simulink model "Project_VirtualWall_V7"  (R2014a)
settings: Solver=FixedStepDiscrete  StartTime=0.0  StopTime=inf  FixedStep=0.0002  RelTol=1e-3
PreLoadFcn:
  | SampleTime = 0.0002;
  | 
  | omega_set = Simulink.Signal;
  | omega_set.Description = ' Omega control set parameter (for read)';
  | omega_set.DataType = 'double';
  | omega_set.Complexity = 'real';
  | omega_set.Dimensions = 9;
  | omega_set.SamplingMode = 'Sample based';
  | omega_set.SampleTime = SampleTime;
  | omega_set.InitialValue = '[0 0 0 0 0 0 0 0 0] ';
undefined symbols (not defined in the file or in its folder): mdionipcie
libraries: slrtlib x16, simulink x9, dsparch4 x6, simulink_extras x3, phantom_kinematics_lib x2, dspmtrx3 x2, dspswit3 x1
settings Model: SimulationMode=external  BufferReuse=off  Creator=janezp  LastModifiedBy=student
settings SolverCC: EnableConcurrentExecution=on
settings DataIOCC: LimitDataPoints=off  MaxDataPoints=5000000  SaveFormat=Structure  SignalLogging=off  SaveTime=off
settings OptimizationCC: BlockReduction=off  OptimizeBlockIOStorage=off  BufferReuse=off  GlobalBufferReuse=off  ExpressionFolding=off  ExpressionDepthLimit=2147483647  LocalBlockOutputs=off  InitFltsAndDblsToZero=on
settings DebuggingCC: SaveWithParameterizedLinksMsg=none  MergeDetectMultiDrivingBlocksExec=error  SignalResolutionControl=TryResolveAllWithWarning  InheritedTsInSrcMsg=none  MultiTaskDSMMsg=warning  MultiTaskCondExecSysMsg=none  UnconnectedInputMsg=none  UnconnectedOutputMsg=none  UnconnectedLineMsg=none  StateNameClashWarn=warning
settings HardwareCC: ProdIntDivRoundTo=Zero  ProdEndianess=LittleEndian  ProdHWDeviceType=Generic->32-bit x86 compatible
settings SFSimCC: SimParseCustomCode=off
settings RTWCC: SystemTargetFile=slrt.tlc  TemplateMakefile=slrt_default_tmf  Description=Simulink Real-Time  ProcessScript=slrt_make_rtw_hook  CustomInclude="\"C:\\Program Files (x86)\\MATLAB\\R2014a\\toolbox\\robotica\\haptics\\collisiondetection\\\""  IncludeERTFirstTime=on  RTWCompilerOptimization=On
settings RTWCC: CustomLibrary=|
  | \..\..\math\mathlib.lib
  | deBug.obj
settings SimulinkRealTimeCC: GeneratePreprocessorConditionals=Disable all  EnableShiftOperators=on  RL32LogBufSizeModifier=5000000

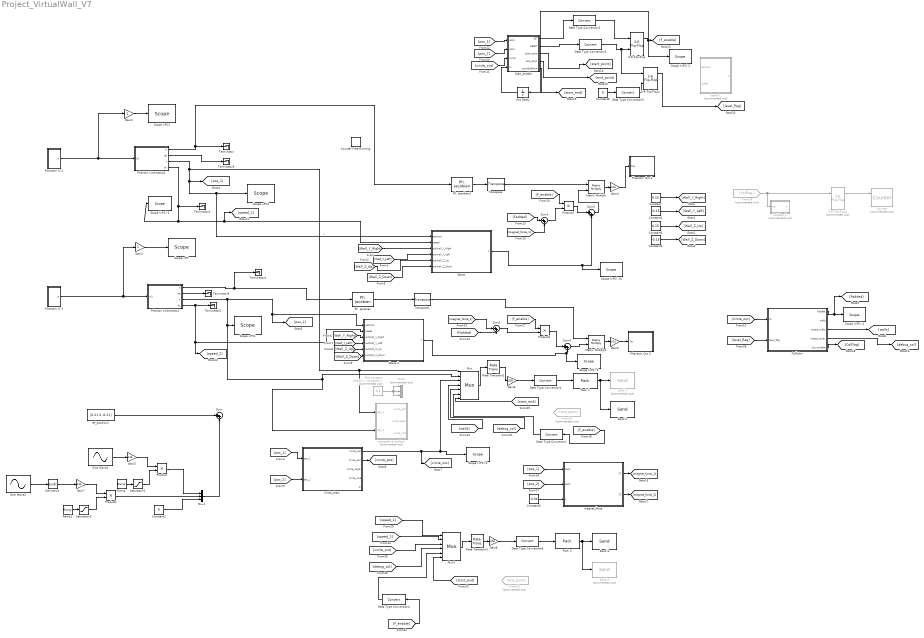
== system Project_VirtualWall_V7 ==
  "Circle_draw " : MATLAB Function  TreatAsAtomicUnit=on
  "Collision " : MATLAB Function  TreatAsAtomicUnit=on
  Collision 1 : MATLAB Function  Commented=on  TreatAsAtomicUnit=on
  Constant : Constant  Value=0.15
  Constant1 : Constant  Value=-0.15
  Constant2 : Constant  Value=0  OutDataTypeStr=double  SampleTime=-1
  Constant3 : Constant  Value=0.15
  Constant4 : Constant  Value=-0.15
  Constant5 : Constant  Value=0.04
  Constant6 : Constant  Value=0
  Counter : dspswit3/Counter  Commented=on  Direction=Up  CountEvent=Rising edge  CounterSize=User defined  MaxCount=255  InitialCount=0  Output=Count and Hit  HitValue=32  ResetInput=on  SamplesPerFrame=1  Ts=1  CntDtype=double  HitDtype=Logical
  Counter Free-Running : simulink/Sources/Counter Free-Running  NumBits=16  tsamp=-1
  Data Type Conversion{,1..6} (7 alike) : DataTypeConversion
  Derivative : Derivative
  From24 : From  Commented=on  GotoTag=ColFlag
  From26 : From  Commented=on  GotoTag=end_point
  From33 : From  Commented=on  GotoTag=end_point
  Gain1 : Gain
  Gain2 : Gain
  Gain3 : Gain  Gain=0.05
  Gain4 : Gain  Gain=0.15
  Gain5 : Gain  Gain=0.15
  Gain6 : Gain  Gain=100
  Gain7 : Gain  Gain=0.05
  Gain8 : Gain  Gain=100
  Matrix Multiply : Product  Multiplication=Matrix(*)
  Matrix Multiply1 : Product  Multiplication=Matrix(*)
  Mux : Mux  Inputs=7
  Mux1 : Mux  Inputs=3
  Mux2 : Mux  Commented=on  Inputs=3
  Mux3 : Mux  Inputs=6
  Pack 1 : slrtlib/UDP/Pack   datatypes={'single'}  byteAlign=1
  Pack 2 : slrtlib/UDP/Pack   datatypes={'single'}  byteAlign=1
  Ph. Jacobian : phantom_kinematics_lib/Ph. Jacobian
  Ph. Jacobian1 : phantom_kinematics_lib/Ph. Jacobian
      link override phantomJacobian: FunctionName=phantomJacobian  SFunctionModules=phantomJacobian_wrapper
  Phantom In 2 : Subsystem  mask(Phantom Input){channel=3, sampletime=0.0002, slot=[2,3], phantomid=Phantom ONE}
      mask prompts: channel "Number of joints:"; sampletime "Sample time:"; slot "PCI slot (-1: autosearch):"; phantomid "Phantom ID:"
      mask help: Block output is a vector of Phantom joint angles.
      mask init:
      | set_param(gcb', 'LinkStatus', 'none')
      | current_block = gcb;
      | 
      | line = find_system(current_block, 'LookUnderMasks', 'on', 'FindAll', 'on', 'type', 'line');
      | for ii=1:length(line)
      |     delete_line(line(ii));
      | end
      | 
      | set_param([current_block,'/Phantom Input'], 'channel', num2str(channel));
      | set_param([current_block,'/Phantom Input'], 'sampletime', sampletime);
      | set_param([current_block,'/Phantom Input'], 'slot', slot);
      | set_param([current_block,'/Phantom Input'], 'phantomid', num2str(phantomid-1));
      | 
      | set_param([current_block,'/Mux'], 'Inputs', int2str(channel)); 
      | 
      | add_line(current_block, 'Mux/1', 'q/1'); 
      | 
      | for i=1:channel,
      |     add_line(current_block, ['Phantom Input/', int2str(i)], ['Mux/', int2str(i)]); 
      | end
      mask TypeOptions phantomid: Phantom ONE | Phantom TWO | Phantom THREE
  Phantom In 3 : Subsystem  mask(Phantom Input){channel=3, sampletime=0.0002, slot=[4,0], phantomid=Phantom TWO}
      mask prompts: channel "Number of joints:"; sampletime "Sample time:"; slot "PCI slot (-1: autosearch):"; phantomid "Phantom ID:"
      mask help: Block output is a vector of Phantom joint angles.
      mask init: same as Project_VirtualWall_V7/Phantom In 2
      mask TypeOptions phantomid: Phantom ONE | Phantom TWO | Phantom THREE
  Phantom Out 2 : Subsystem  mask(Phantom Output){sampletime=0.0002, slot=[2,3]}
      mask prompts: sampletime "Sample time:"; slot "PCI slot (-1: autosearch):"
      mask help: Input is torque vector for Phantom motors.
      mask init:
      | set_param(gcb', 'LinkStatus', 'none')
      | current_block = gcb;
      | 
      | set_param([current_block,'/Phantom Output'], 'sampletime', sampletime);
      | set_param([current_block,'/Phantom Output'], 'slot', slot);
  Phantom Out 3 : Subsystem  mask(Phantom Output){sampletime=0.0002, slot=[4,0]}
      mask prompts: sampletime "Sample time:"; slot "PCI slot (-1: autosearch):"
      mask help: Input is torque vector for Phantom motors.
      mask init:
      | set_param(gcb', 'LinkStatus', 'none')
      | current_block = gcb;
      | 
      | set_param([current_block,'/Phantom Output'], 'sampletime', sampletime);
      | set_param([current_block,'/Phantom Output'], 'slot', slot);
  Phanton kinematics1 : Subsystem
  Phanton kinematics2 : Subsystem
  Product{,1..3} (4 alike) : Product
  Ramp : simulink/Sources/Ramp  slope=0.25  start=1  X0=0
  Ramp1 : simulink/Sources/Ramp  slope=0.25  start=1  X0=0
  Rate Transition1 : RateTransition  OutPortSampleTime=0.01
  Rate Transition2 : RateTransition  OutPortSampleTime=0.01
  S-R Flip-Flop : simulink_extras/Flip Flops/S-R Flip-Flop  initial_condition=0
  S-R Flip-Flop1 : simulink_extras/Flip Flops/S-R Flip-Flop  Commented=on  initial_condition=0
  S-R Flip-Flop2 : simulink_extras/Flip Flops/S-R Flip-Flop  initial_condition=0
  Saturation1 : Saturate  UpperLimit=1  LowerLimit=0
  Saturation2 : Saturate  UpperLimit=1  LowerLimit=0
  Scope (xPC) 1 : slrtlib/Displays and Logging/Scope   scopeno=6  scopetype=Target  autostart=on  viewmode=Numerical  formatstr='Tx: %15.6f, Ty: %15.6f, Tz: %15.6f'  grid=on  ylimits=[0,0]  nosamples=50  noprepostsamples=0  interleave=1  triggermode=FreeRun  triggersignal=1  trigsignalfromport=off  triggerlevel=0.0  triggerslope=Either  triggerscope=1  triggersample=0  filename=data.dat  mode=Lazy  writesize=512  autorestart=off  dynamicfilemode=off  maxwritefilesize=512*1024^2
  Scope (xPC) 10 : slrtlib/Displays and Logging/Scope   scopeno=10  scopetype=Target  autostart=on  viewmode=Numerical  formatstr='Fx1: %15.6f,Fy: %15.6f,Fz: %15.6f'  grid=on  ylimits=[0,0]  nosamples=50  noprepostsamples=0  interleave=1  triggermode=FreeRun  triggersignal=1  trigsignalfromport=off  triggerlevel=0.0  triggerslope=Either  triggerscope=1  triggersample=0  filename=data.dat  mode=Lazy  writesize=512  autorestart=off  dynamicfilemode=off  maxwritefilesize=512*1024^2
  Scope (xPC) 2 : slrtlib/Displays and Logging/Scope   scopeno=5  scopetype=Target  autostart=on  viewmode=Numerical  formatstr='Fx1: %15.6f,Fy: %15.6f,Fz: %15.6f'  grid=on  ylimits=[0,0]  nosamples=50  noprepostsamples=0  interleave=1  triggermode=FreeRun  triggersignal=1  trigsignalfromport=off  triggerlevel=0.0  triggerslope=Either  triggerscope=1  triggersample=0  filename=data.dat  mode=Lazy  writesize=512  autorestart=off  dynamicfilemode=off  maxwritefilesize=512*1024^2
  Scope (xPC) 3 : slrtlib/Displays and Logging/Scope   scopeno=7  scopetype=Target  autostart=on  viewmode=Numerical  formatstr='Fx1: %15.6f,Fy: %15.6f,Fz: %15.6f'  grid=on  ylimits=[0,0]  nosamples=50  noprepostsamples=0  interleave=1  triggermode=FreeRun  triggersignal=1  trigsignalfromport=off  triggerlevel=0.0  triggerslope=Either  triggerscope=1  triggersample=0  filename=data.dat  mode=Lazy  writesize=512  autorestart=off  dynamicfilemode=off  maxwritefilesize=512*1024^2
  Scope (xPC) 4 : slrtlib/Displays and Logging/Scope   scopeno=8  scopetype=Target  autostart=on  viewmode=Numerical  formatstr='Fx1: %15.6f,Fy: %15.6f,Fz: %15.6f'  grid=on  ylimits=[0,0]  nosamples=50  noprepostsamples=0  interleave=1  triggermode=FreeRun  triggersignal=1  trigsignalfromport=off  triggerlevel=0.0  triggerslope=Either  triggerscope=1  triggersample=0  filename=data.dat  mode=Lazy  writesize=512  autorestart=off  dynamicfilemode=off  maxwritefilesize=512*1024^2
  Scope (xPC) 5 : slrtlib/Displays and Logging/Scope   scopeno=9  scopetype=Target  autostart=on  viewmode=Numerical  formatstr='Fx1: %15.6f,Fy: %15.6f,Fz: %15.6f'  grid=on  ylimits=[0,0]  nosamples=50  noprepostsamples=0  interleave=1  triggermode=FreeRun  triggersignal=1  trigsignalfromport=off  triggerlevel=0.0  triggerslope=Either  triggerscope=1  triggersample=0  filename=data.dat  mode=Lazy  writesize=512  autorestart=off  dynamicfilemode=off  maxwritefilesize=512*1024^2
  Scope xPC : slrtlib/Displays and Logging/Scope   scopeno=1  scopetype=Target  autostart=on  viewmode=Numerical  formatstr='q1r1: %15.6f,q2r1: %15.6f,q3r1: %15.6f'  grid=on  ylimits=[0,0]  nosamples=250  noprepostsamples=0  interleave=1  triggermode=FreeRun  triggersignal=1  trigsignalfromport=off  triggerlevel=0.0  triggerslope=Either  triggerscope=1  triggersample=0  filename=data.dat  mode=Lazy  writesize=512  autorestart=off  dynamicfilemode=off  maxwritefilesize=512*1024^2
  Scope xPC1 : slrtlib/Displays and Logging/Scope   scopeno=2  scopetype=Target  autostart=on  viewmode=Numerical  formatstr='Xr1: %15.6f, Yr1: %15.6f, Zr1: %15.6f'  grid=on  ylimits=[0,0]  nosamples=250  noprepostsamples=0  interleave=1  triggermode=FreeRun  triggersignal=1  trigsignalfromport=off  triggerlevel=0.0  triggerslope=Either  triggerscope=1  triggersample=0  filename=data.dat  mode=Lazy  writesize=512  autorestart=off  dynamicfilemode=off  maxwritefilesize=512*1024^2
  Scope xPC2 : slrtlib/Displays and Logging/Scope   scopeno=3  scopetype=Target  autostart=on  viewmode=Numerical  formatstr='q1r1: %15.6f,q2r1: %15.6f,q3r1: %15.6f'  grid=on  ylimits=[0,0]  nosamples=250  noprepostsamples=0  interleave=1  triggermode=FreeRun  triggersignal=1  trigsignalfromport=off  triggerlevel=0.0  triggerslope=Either  triggerscope=1  triggersample=0  filename=data.dat  mode=Lazy  writesize=512  autorestart=off  dynamicfilemode=off  maxwritefilesize=512*1024^2
  Scope xPC3 : slrtlib/Displays and Logging/Scope   scopeno=4  scopetype=Target  autostart=on  viewmode=Numerical  formatstr='Xr1: %15.6f, Yr1: %15.6f, Zr1: %15.6f'  grid=on  ylimits=[0,0]  nosamples=250  noprepostsamples=0  interleave=1  triggermode=FreeRun  triggersignal=1  trigsignalfromport=off  triggerlevel=0.0  triggerslope=Either  triggerscope=1  triggersample=0  filename=data.dat  mode=Lazy  writesize=512  autorestart=off  dynamicfilemode=off  maxwritefilesize=512*1024^2
  Send 1 : slrtlib/UDP/Send   Commented=on  ipAddress=192.168.65.34  ipPort=25008  localPort=-1  vblLen=off  sampletime=0.01
  Send 2 : slrtlib/UDP/Send   ipAddress=192.168.65.35  ipPort=25008  localPort=-1  vblLen=off  sampletime=0.01
  Send 3 : slrtlib/UDP/Send   ipAddress=192.168.65.34  ipPort=25008  localPort=-1  vblLen=off  sampletime=0.01
  Send 4 : slrtlib/UDP/Send   Commented=on  ipAddress=192.168.65.35  ipPort=25008  localPort=-1  vblLen=off  sampletime=0.01
  Sine Wave1 : Sin  SineType=Sample based  Samples=50000  SampleTime=1/5000
  Sine Wave2 : Sin  SineType=Sample based  Samples=50000  SampleTime=1/5000
  "Start_enable " : MATLAB Function  TreatAsAtomicUnit=on
  "Stena " : MATLAB Function  TreatAsAtomicUnit=on
  Stena 1 : MATLAB Function  Commented=on  TreatAsAtomicUnit=on
  Stena 2 : MATLAB Function  TreatAsAtomicUnit=on
  Sum{,1..4} (5 alike) : Sum  Inputs=|++
  Terminator{,1..5} (6 alike) : Terminator
  Test constant (checking connection) : Constant  Commented=on  Value=0.2  SampleTime=0.01
  Transpose : dspmtrx3/Transpose  Hermitian=off  overflowFlag=off
  Transpose1 : dspmtrx3/Transpose  Hermitian=off  overflowFlag=off
  Unit Delay : UnitDelay  SampleTime=-1
  cooperative position : MATLAB Function  Commented=on  TreatAsAtomicUnit=on
  magnet_force : MATLAB Function  TreatAsAtomicUnit=on
  ref_position2 : Constant  Value=[0.21 0 -0.21]
  wires:
  Gain1/1 -> Scope xPC/1
  Phanton kinematics1/4(dx) -> [speed_2], Stena 2/2(speed), Terminator2/1
  Phantom In 3/1(q) -> Phanton kinematics1/1(In1), Gain1/1
  Gain2/1 -> Scope xPC2/1
  Phantom In 2/1(q) -> Gain2/1, Phanton kinematics2/1(In1)
  Phanton kinematics2/3(x) -> [pos_1], "Stena "/1(position), Scope xPC3/1, cooperative position/1(pos_1), Mux/1  "x"
  Phanton kinematics1/3(x) -> [pos_2], Stena 2/1(position), cooperative position/2(pos_2), Mux/2, Scope xPC1/1
  Pack 1/1 -> Send 2/1, Send 1/1
  Data Type Conversion1/1 -> Pack 1/1
  Rate Transition1/1 -> Gain6/1
  Mux/1 -> Rate Transition1/1
  Gain3/1 -> Product/1
  Ramp/1 -> Saturation1/1
  Sine Wave1/1 -> Gain3/1
  Product/1 -> Mux1/1
  Gain7/1 -> Product1/1
  Ramp1/1 -> Saturation2/1
  Product1/1 -> Mux1/2
  Derivative/1 -> Gain7/1
  Constant2/1 -> Mux1/3
  Saturation1/1 -> Product/2
  Saturation2/1 -> Product1/2
  Sine Wave2/1 -> Derivative/1
  ref_position2/1 -> Sum/1
  Mux1/1 -> Sum/2
  Phanton kinematics2/1(q) -> Ph. Jacobian1/1, Terminator/1
  Phanton kinematics2/2(dq) -> Terminator3/1
  Ph. Jacobian1/1 -> Transpose/1
  Transpose/1 -> Matrix Multiply/1
  Gain4/1 -> Phantom Out 2/1(Tau)
  Phanton kinematics1/1(q) -> Ph. Jacobian/1, Terminator4/1
  Phanton kinematics1/2(dq) -> Terminator5/1
  Ph. Jacobian/1 -> Transpose1/1
  Gain5/1 -> Phantom Out 3/1(Tau)
  Transpose1/1 -> Matrix Multiply1/1
  Stena 2/1(T) -> Scope (xPC) 5/1, Sum4/2
  Gain6/1 -> Data Type Conversion1/1
  Test constant (checking connection)/1 -> Mux2/3, Mux2/2, Mux2/1
  Constant/1 -> [Wall_Y_Right]
  Constant1/1 -> [Wall_Y_Left]
  Constant3/1 -> [Wall_Z_Up]
  Constant4/1 -> [Wall_Z_Down]
  [Wall_Y_Right] -> "Stena "/3(outWall_Y_Right)
  [Wall_Y_Left] -> "Stena "/4(outWall_Y_Left)
  [Wall_Z_Up] -> "Stena "/5(outWall_Z_Up)
  [Wall_Z_Down] -> "Stena "/6(outWall_Z_Down)
  "Stena "/1(T) -> Sum3/2, Scope (xPC) 10/1
  [pos_1] -> "Circle_draw "/1(pos_1)
  [pos_2] -> "Circle_draw "/2(pos_2)
  "Circle_draw "/1(circle_out) -> [circle_out], Scope (xPC) 3/1, Mux/3
  [Wall_Y_Right] -> Stena 2/3(outWall_Y_Right)
  [Wall_Y_Left] -> Stena 2/4(outWall_Y_Left)
  [Wall_Z_Up] -> Stena 2/5(outWall_Z_Up)
  [Wall_Z_Down] -> Stena 2/6(outWall_Z_Down)
  "Circle_draw "/2(circle_pos) -> [circle_pos]
  [circle_out] -> "Collision "/1(cir)
  "Collision "/3(output_walls) -> [walls]
  [walls] -> Mux/4
  "Collision "/1(Fadded) -> [Fadded], Scope (xPC) 4/1
  [Fadded] -> Sum1/1
  [Fadded] -> Sum2/2
  "Collision "/4(output_array) -> [debug_col]
  [debug_col] -> Mux/5
  Phanton kinematics2/4(dx) -> Scope (xPC) 1/1, [speed_1], "Stena "/2(speed), Terminator1/1
  [pos_1] -> magnet_force/1(pos1)
  [pos_2] -> magnet_force/2(pos2)
  [F_enable] -> Product2/1
  [circle_out] -> "Start_enable "/3(circle)
  [pos_2] -> "Start_enable "/2(pos2)
  [pos_1] -> "Start_enable "/1(pos1)
  "Start_enable "/3(start_point) -> [start_point]
  [start_end] -> Mux/7
  S-R Flip-Flop/1 -> Scope (xPC) 2/1, [F_enable], Unit Delay/1
  "Start_enable "/4(end_point) -> [end_point]
  Constant5/1 -> magnet_force/3(L)
  Data Type Conversion/1 -> Mux/6
  [F_enable] -> Data Type Conversion/1
  magnet_force/2(F2) -> [magnet_force_2]
  magnet_force/1(F1) -> [magnet_force_1]
  [magnet_force_2] -> Sum2/1
  S-R Flip-Flop1/1 -> Counter/1
  "Collision "/5(col_variable) -> [ColFlag]
  From24/1 -> Collision 1/1(out), S-R Flip-Flop1/1
  Sum1/1 -> Product2/2
  "Start_enable "/1(SET) -> Data Type Conversion2/1
  Data Type Conversion2/1 -> S-R Flip-Flop/1
  "Start_enable "/2(RESET) -> Data Type Conversion3/1
  Data Type Conversion3/1 -> S-R Flip-Flop2/1, S-R Flip-Flop/2
  [F_enable] -> Product3/1
  Sum2/1 -> Product3/2
  "Start_enable "/5(startEndPoint) -> [start_end]
  Constant6/1 -> Data Type Conversion5/1
  Data Type Conversion5/1 -> S-R Flip-Flop2/2
  Unit Delay/1 -> "Start_enable "/4(in)
  S-R Flip-Flop2/1 -> [level_flag]
  [level_flag] -> "Collision "/2(level_flag)
  Matrix Multiply1/1 -> Gain5/1
  Sum4/1 -> Matrix Multiply1/2
  Product3/1 -> Sum4/1
  Matrix Multiply/1 -> Gain4/1
  Product2/1 -> Sum3/1
  Sum3/1 -> Matrix Multiply/2
  [magnet_force_1] -> Sum1/2
  Pack 2/1 -> Send 4/1, Send 3/1
  Data Type Conversion6/1 -> Pack 2/1
  Rate Transition2/1 -> Gain8/1
  Mux3/1 -> Rate Transition2/1
  Gain8/1 -> Data Type Conversion6/1
  [F_enable] -> Data Type Conversion4/1
  [speed_1] -> Mux3/1
  [speed_2] -> Mux3/2
  [circle_out] -> Mux3/3
  [debug_col] -> Mux3/4
  Data Type Conversion4/1 -> Mux3/5
  [start_end] -> Mux3/6

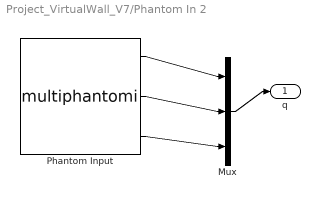
== system Project_VirtualWall_V7/Phantom In 2 ==
  Mux : Mux  Inputs=3
  Phantom Input : S-Function  InitFcn=mdionipcie(1);  FunctionName=multiphantomi  Parameters=channel, sampletime, slot, phantomid  EnableBusSupport=off  mask(Phantom Input){channel=3, sampletime=0.0002, slot=[2,3], phantomid=0}
      mask prompts: channel "Number of joints:"; sampletime "Sample time:"; slot "PCI slot (-1: autosearch):"; phantomid "Phantom ID"
      mask Display: disp('Phantom Input');
  q : Outport
  wires:
  Mux/1 -> q/1
  Phantom Input/1 -> Mux/1
  Phantom Input/2 -> Mux/2
  Phantom Input/3 -> Mux/3

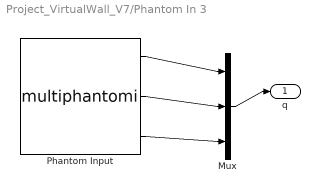
== system Project_VirtualWall_V7/Phantom In 3 ==
  Mux : Mux  Inputs=3
  Phantom Input : S-Function  InitFcn=mdionipcie(1);  FunctionName=multiphantomi  Parameters=channel, sampletime, slot, phantomid  EnableBusSupport=off  mask(Phantom Input){channel=3, sampletime=0.0002, slot=[4,0], phantomid=1}
      mask prompts: channel "Number of joints:"; sampletime "Sample time:"; slot "PCI slot (-1: autosearch):"; phantomid "Phantom ID"
      mask Display: disp('Phantom Input');
  q : Outport
  wires:
  Mux/1 -> q/1
  Phantom Input/1 -> Mux/1
  Phantom Input/2 -> Mux/2
  Phantom Input/3 -> Mux/3

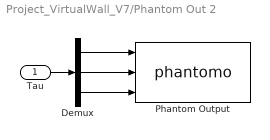
== system Project_VirtualWall_V7/Phantom Out 2 ==
  Tau : Inport
  Demux : Demux  Outputs=3
  Phantom Output : S-Function  InitFcn=mdionipcie(1);  FunctionName=phantomo  Parameters="channel,  reset, initValue, sampletime,slot, control, boardType"  EnableBusSupport=off  mask(Phantom Output){channel=[1 1 1], sampletime=0.0002, slot=[2,3]}
      mask prompts: channel "Channel vector:"; sampletime "Sample time:"; slot "PCI slot (-1: autosearch):"
      mask init:
      | control=0;
      | boardType=21;
      | initValue=[0 0 0];
      | reset=[1];
      mask Display: disp('Phantom \n Output');port_label('input',1,'Tau1');port_label('input',2,'Tau2');port_label('input',3,'Tau3');
  wires:
  Demux/1 -> Phantom Output/1
  Demux/2 -> Phantom Output/2
  Demux/3 -> Phantom Output/3
  Tau/1 -> Demux/1

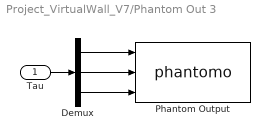
== system Project_VirtualWall_V7/Phantom Out 3 ==
  Tau : Inport
  Demux : Demux  Outputs=3
  Phantom Output : S-Function  InitFcn=mdionipcie(1);  FunctionName=phantomo  Parameters="channel,  reset, initValue, sampletime,slot, control, boardType"  EnableBusSupport=off  mask(Phantom Output){channel=[1 1 1], sampletime=0.0002, slot=[4,0]}
      mask prompts: channel "Channel vector:"; sampletime "Sample time:"; slot "PCI slot (-1: autosearch):"
      mask init:
      | control=0;
      | boardType=21;
      | initValue=[0 0 0];
      | reset=[1];
      mask Display: disp('Phantom \n Output');port_label('input',1,'Tau1');port_label('input',2,'Tau2');port_label('input',3,'Tau3');
  wires:
  Tau/1 -> Demux/1
  Demux/3 -> Phantom Output/3
  Demux/2 -> Phantom Output/2
  Demux/1 -> Phantom Output/1

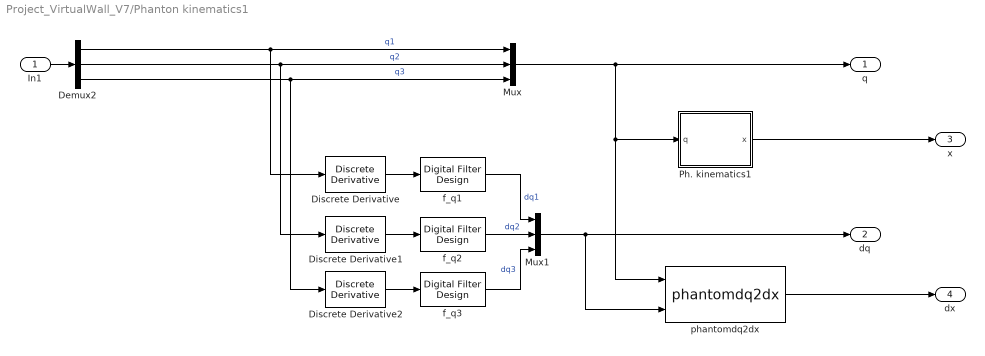
== system Project_VirtualWall_V7/Phanton kinematics1 ==
  In1 : Inport
  Demux2 : Demux  Outputs=3
  Discrete Derivative : simulink/Discrete/Discrete Derivative  gainval=1.0  ICPrevScaledInput=0.0  OutMin=[]  OutMax=[]  OutDataType=sfix(16)  OutScaling=2^-10  DoSatur=off
  Discrete Derivative1 : simulink/Discrete/Discrete Derivative  gainval=1.0  ICPrevScaledInput=0.0  OutMin=[]  OutMax=[]  OutDataType=sfix(16)  OutScaling=2^-10  DoSatur=off
  Discrete Derivative2 : simulink/Discrete/Discrete Derivative  gainval=1.0  ICPrevScaledInput=0.0  OutMin=[]  OutMax=[]  OutDataType=sfix(16)  OutScaling=2^-10  DoSatur=off
  Mux : Mux  Inputs=3
  Mux1 : Mux  Inputs=3
  Ph. kinematics1 : Subsystem  AncestorBlock=phantom_kinematics_lib/Ph. kinematics  mask(Phantom direct kinematics){}
      mask help:
      | Phantom direct kinematic model
      | q - joint angles
      | x - ned-effector position
  f_q1 : dsparch4/Digital Filter Design  mwdsp_browser_bugfix_var=off
  f_q2 : dsparch4/Digital Filter Design  mwdsp_browser_bugfix_var=off
  f_q3 : dsparch4/Digital Filter Design  mwdsp_browser_bugfix_var=off
  phantomdq2dx : S-Function  InitFcn=try, set_param(gcb,'FunctionName','phantomdq2dx'), end  FunctionName=phantomdq2dx  SFunctionModules=phantomdq2dx_wrapper  EnableBusSupport=off  mask(S-Function Builder){}
      mask help: The S-Function Builder block creates a wrapper C-MEX S-function from your supplied C code with multiple input ports, output ports, and a variable number of scalar, vector, or matrix parameters. The input and output ports can propagate Simulink built-in data types, fixed-point datatypes, complex, frame, 1-D, and 2-D signals. This block also supports discrete and continuous states of type real. You can optionally have the block generate a TLC file to be used with Real-Time Workshop for code generation.
      mask init:
      | val = [[.9  0.75 0.75 1 1 .9 .9 1]',[1 1 0.75 0.75 .9 .9 1 .9]'];try , sys = get_param(gcb,'SfunBuilderFcnName');if isempty(sys), sys = get_param(gcb,'FunctionName'); end,catch, sys = get_param(gcb,'FunctionName'); end
      settings: CopyFcn=set_param(gcbh,'LinkStatus','none')  PreSaveFcn=try, set_param(gcb,'FunctionName','phantomdq2dx'), end  OpenFcn=sfunctionwizard(gcbh)
      mask Display: plot(val(:,1),val(:,2)),disp(sys), port_label('input',1,'q'), port_label('input',2,'dq'), port_label('output',1,'dx')
  q : Outport
  dq : Outport  Port=2
  x : Outport  Port=3
  dx : Outport  Port=4
  wires:
  In1/1 -> Demux2/1
  Ph. kinematics1/1(x) -> x/1
  phantomdq2dx/1 -> dx/1
  f_q3/1 -> Mux1/3  "dq3"
  f_q2/1 -> Mux1/2  "dq2"
  Mux1/1 -> phantomdq2dx/2, dq/1
  Discrete Derivative2/1 -> f_q3/1
  Discrete Derivative1/1 -> f_q2/1
  f_q1/1 -> Mux1/1  "dq1"
  Discrete Derivative/1 -> f_q1/1
  Mux/1 -> Ph. kinematics1/1(q), phantomdq2dx/1, q/1
  Demux2/3 -> Mux/3, Discrete Derivative2/1  "q3"
  Demux2/2 -> Mux/2, Discrete Derivative1/1  "q2"
  Demux2/1 -> Mux/1, Discrete Derivative/1  "q1"

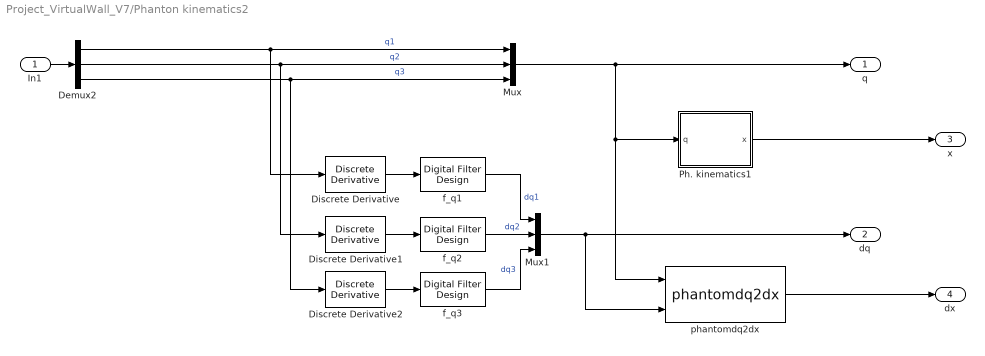
== system Project_VirtualWall_V7/Phanton kinematics2 ==
  In1 : Inport
  Demux2 : Demux  Outputs=3
  Discrete Derivative : simulink/Discrete/Discrete Derivative  gainval=1.0  ICPrevScaledInput=0.0  OutMin=[]  OutMax=[]  OutDataType=sfix(16)  OutScaling=2^-10  DoSatur=off
  Discrete Derivative1 : simulink/Discrete/Discrete Derivative  gainval=1.0  ICPrevScaledInput=0.0  OutMin=[]  OutMax=[]  OutDataType=sfix(16)  OutScaling=2^-10  DoSatur=off
  Discrete Derivative2 : simulink/Discrete/Discrete Derivative  gainval=1.0  ICPrevScaledInput=0.0  OutMin=[]  OutMax=[]  OutDataType=sfix(16)  OutScaling=2^-10  DoSatur=off
  Mux : Mux  Inputs=3
  Mux1 : Mux  Inputs=3
  Ph. kinematics1 : Subsystem  AncestorBlock=phantom_kinematics_lib/Ph. kinematics  mask(Phantom direct kinematics){}
      mask help:
      | Phantom direct kinematic model
      | q - joint angles
      | x - ned-effector position
  f_q1 : dsparch4/Digital Filter Design  mwdsp_browser_bugfix_var=off
  f_q2 : dsparch4/Digital Filter Design  mwdsp_browser_bugfix_var=off
  f_q3 : dsparch4/Digital Filter Design  mwdsp_browser_bugfix_var=off
  phantomdq2dx : S-Function  InitFcn=try, set_param(gcb,'FunctionName','phantomdq2dx'), end  FunctionName=phantomdq2dx  SFunctionModules=phantomdq2dx_wrapper  EnableBusSupport=off  mask(S-Function Builder){}
      mask help: The S-Function Builder block creates a wrapper C-MEX S-function from your supplied C code with multiple input ports, output ports, and a variable number of scalar, vector, or matrix parameters. The input and output ports can propagate Simulink built-in data types, fixed-point datatypes, complex, frame, 1-D, and 2-D signals. This block also supports discrete and continuous states of type real. You can optionally have the block generate a TLC file to be used with Real-Time Workshop for code generation.
      mask init: same as Project_VirtualWall_V7/Phanton kinematics1/phantomdq2dx
      settings: CopyFcn=set_param(gcbh,'LinkStatus','none')  PreSaveFcn=try, set_param(gcb,'FunctionName','phantomdq2dx'), end  OpenFcn=sfunctionwizard(gcbh)
      mask Display: plot(val(:,1),val(:,2)),disp(sys), port_label('input',1,'q'), port_label('input',2,'dq'), port_label('output',1,'dx')
  q : Outport
  dq : Outport  Port=2
  x : Outport  Port=3
  dx : Outport  Port=4
  wires:
  Demux2/1 -> Discrete Derivative/1, Mux/1  "q1"
  Demux2/2 -> Discrete Derivative1/1, Mux/2  "q2"
  Demux2/3 -> Discrete Derivative2/1, Mux/3  "q3"
  Mux/1 -> q/1, phantomdq2dx/1, Ph. kinematics1/1(q)
  Discrete Derivative/1 -> f_q1/1
  f_q1/1 -> Mux1/1  "dq1"
  Discrete Derivative1/1 -> f_q2/1
  Discrete Derivative2/1 -> f_q3/1
  Mux1/1 -> dq/1, phantomdq2dx/2
  f_q2/1 -> Mux1/2  "dq2"
  f_q3/1 -> Mux1/3  "dq3"
  phantomdq2dx/1 -> dx/1
  Ph. kinematics1/1(x) -> x/1
  In1/1 -> Demux2/1

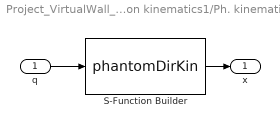
== system Project_VirtualWall_V7/Phanton kinematics1/Ph. kinematics1 ==
  q : Inport
  S-Function Builder : S-Function  InitFcn=try, set_param(gcb,'FunctionName','phantomDirKin'), end  FunctionName=phantomDirKin  SFunctionModules=phantomDirKin_wrapper  EnableBusSupport=off  mask(S-Function Builder){}
      mask help: The S-Function Builder block creates a wrapper C-MEX S-function from your supplied C code with multiple input ports, output ports, and a variable number of scalar, vector, or matrix parameters. The input and output ports can propagate Simulink built-in data types, fixed-point datatypes, complex, frame, 1-D, and 2-D signals. This block also supports discrete and continuous states of type real. You can optionally have the block generate a TLC file to be used with Real-Time Workshop for code generation.
      mask init: same as Project_VirtualWall_V7/Phanton kinematics1/phantomdq2dx
      settings: CopyFcn=set_param(gcbh,'LinkStatus','none')  PreSaveFcn=try, set_param(gcb,'FunctionName','phantomDirKin'), end  OpenFcn=sfunctionwizard(gcbh)
      mask Display: plot(val(:,1),val(:,2)),disp(sys), port_label('input',1,'q'), port_label('output',1,'x')
  x : Outport
  wires:
  q/1 -> S-Function Builder/1
  S-Function Builder/1 -> x/1

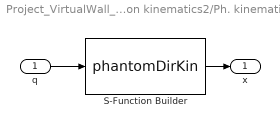
== system Project_VirtualWall_V7/Phanton kinematics2/Ph. kinematics1 ==
  q : Inport
  S-Function Builder : S-Function  InitFcn=try, set_param(gcb,'FunctionName','phantomDirKin'), end  FunctionName=phantomDirKin  SFunctionModules=phantomDirKin_wrapper  EnableBusSupport=off  mask(S-Function Builder){}
      mask help: The S-Function Builder block creates a wrapper C-MEX S-function from your supplied C code with multiple input ports, output ports, and a variable number of scalar, vector, or matrix parameters. The input and output ports can propagate Simulink built-in data types, fixed-point datatypes, complex, frame, 1-D, and 2-D signals. This block also supports discrete and continuous states of type real. You can optionally have the block generate a TLC file to be used with Real-Time Workshop for code generation.
      mask init: same as Project_VirtualWall_V7/Phanton kinematics1/phantomdq2dx
      settings: CopyFcn=set_param(gcbh,'LinkStatus','none')  PreSaveFcn=try, set_param(gcb,'FunctionName','phantomDirKin'), end  OpenFcn=sfunctionwizard(gcbh)
      mask Display: plot(val(:,1),val(:,2)),disp(sys), port_label('input',1,'q'), port_label('output',1,'x')
  x : Outport
  wires:
  S-Function Builder/1 -> x/1
  q/1 -> S-Function Builder/1

== matlab function Project_VirtualWall_V7/Stena 2 ==
  data: position input; speed input; T output; outWall_Y_Right input; outWall_Y_Left input; outWall_Z_Up input; outWall_Z_Down input
function T  = control(position, speed, outWall_Y_Right, outWall_Y_Left, outWall_Z_Up, outWall_Z_Down)
%outWall should be outer wall parameters, typically |0.15|. right and up is
%positive while left and down is negative

F= [0; 0; 0];
%Fzac = [0; 0; 0];

%ref pozicija in ravnina
ref_pos=[0.214; 0; -0.21];
% x is always ON
Fzac = ([600; 0; 0].*(ref_pos-position)) - ([10; 3; 3].*(speed));


%F= k(ps-pp)-bv

yWall_R = outWall_Y_Right; %0.15;
yWall_L = outWall_Y_Left; %-0.15;
zWall_U = outWall_Z_Up; %0.15;
zWall_D = outWall_Z_Down; %-0.15;

k=1500;
bforward=10;
max_force=25;
%Y-Walls
if (position(2)>yWall_R)
    if(speed(2) > 0)
        F(2) = max([-max_force; -k * (position(2)-yWall_R) + bforward * speed(2)]);
    else
        F(2) = max([-max_force; -k * (position(2)-yWall_R)]);
    end
elseif (position(2)<yWall_L)
    if(speed(2) < 0)
        F(2) = min([max_force; -k * (position(2)-yWall_L) + bforward * speed(2)]);
    else
        F(2) = min([max_force; -k * (position(2)-yWall_L)]);
    end
else
    F(2)=0 ;
end

%Z-walls
if (position(3)<zWall_D)
    if(speed(3) < 0)
        F(3) = min([max_force; -k * (position(3)-zWall_D) + bforward * speed(3)]);
    else
        F(3) = min([max_force; -k * (position(3)-zWall_D)]);
    end
elseif (position(3)>zWall_U)
    if(speed(3) > 0)
        F(3) = max([-max_force; -k * (position(3)-zWall_U) + bforward * speed(3)]);
    else
        F(3) = max([-max_force; -k * (position(3)-zWall_U)]);
    end
else
    F(3)=0;
end

T=F+Fzac;

== matlab function Project_VirtualWall_V7/magnet_force ==
  data: pos1 input; pos2 input; L input; F1 output; F2 output
function [F1, F2]  = magnet(pos1, pos2,L)
%outWall should be outer wall parameters, typically |0.15|. right and up is
%positive while left and down is negative
k=200;
F1 = [0;0;0];
F2 = [0;0;0];
%unit(pos2-pos1)
F1 = k * (norm(pos2-pos1)-L) * ((pos2-pos1)/norm(pos2-pos1))
%where unit is meant to be the function that outputs the unit vetor that points in the direction of the input vector, and where L is an equilibrium distance between spheres that we change, and k is the spring constant
%for the other sphere, its symmetric
F2= k * (norm(pos1-pos2)-L) * ((pos1-pos2)/norm(pos1-pos2))

== matlab function Project_VirtualWall_V7/Circle_draw  ==
  data: pos_1 input; pos_2 input; circle_out output; circle_pos output; circle_angle output; circle_size output; R output
function [circle_out,circle_pos,circle_angle,circle_size,R] = circle_draw1(pos_1,pos_2)  
    %pos_1 and 2 are the vectors with the x z y positions of the players,
    %circle_angle is in radians cause why not
    % i am assuming pos_2 is the one who starts on the right
    
    pos_1_yz=pos_1([2 3]);
    pos_2_yz=pos_2([2 3]);
    %circle_pos=(pos_1_yz+pos_2_yz)/2; %vector of dimension 2
    circle_pos = [(pos_1(2)-((pos_1(2)-pos_2(2))/2)), (pos_1(3)-((pos_1(3)-pos_2(3))/2))];
    pos_aux=pos_2_yz-pos_1_yz;
    %dx=(pos_1(2)-pos_2(2));
    %dy
    %circle_size=norm(abs((pos_1(2)-pos_2(2))));
    circle_size= norm(pos_1_yz-pos_2_yz);
    R = circle_size/2;
    
    %ANGLE
    circle_angle=atan2(pos_aux(2),pos_aux(1));
    %circle_angle_degree = circle_angle*180/pi;
    % dot1 and dot2 are two points represented as row vectors [x, y]

    % Calculate the vectors from the origin to the dots
    %vec1 = pos_1 - [0, 0];
    %vec2 = pos_2 - [0, 0];
    % Calculate the dot product of the two vectors
    %dot_product = dot(vec1, vec2);
    % Calculate the magnitudes of the vectors
    %magnitude1 = norm(vec1);
    %magnitude2 = norm(vec2);
    % Calculate the cosine of the angle between the vectors
    %cosine_angle = dot_product / (magnitude1 * magnitude2);
    % Calculate the angle in radians using the arccosine function
    %circle_angle = acos(cosine_angle);
    
   
    circle_out = [circle_pos(1),circle_pos(2),circle_size,circle_angle];

== matlab function Project_VirtualWall_V7/Stena  ==
  data: position input; speed input; T output; outWall_Y_Right input; outWall_Y_Left input; outWall_Z_Up input; outWall_Z_Down input
function T  = control(position, speed, outWall_Y_Right, outWall_Y_Left, outWall_Z_Up, outWall_Z_Down)
%outWall should be outer wall parameters, typically |0.15|. right and up is
%positive while left and down is negative

F= [0; 0; 0];
%Fzac = [0; 0; 0];

%ref pozicija in ravnina
ref_pos=[0.205; 0; -0.21];
% x is always ON
Fzac = ([600; 0; 0].*(ref_pos-position)) - ([10; 3; 3].*(speed));


%F= k(ps-pp)-bv

yWall_R = outWall_Y_Right; %0.15;
yWall_L = outWall_Y_Left; %-0.15;
zWall_U = outWall_Z_Up; %0.15;
zWall_D = outWall_Z_Down; %-0.15;

k=1500;
bforward=10;
max_force=25;
%Y-Walls
if (position(2)>yWall_R)
    if(speed(2) > 0)
        F(2) = max([-max_force; -k * (position(2)-yWall_R) + bforward * speed(2)]);
    else
        F(2) = max([-max_force; -k * (position(2)-yWall_R)]);
    end
elseif (position(2)<yWall_L)
    if(speed(2) < 0)
        F(2) = min([max_force; -k * (position(2)-yWall_L) + bforward * speed(2)]);
    else
        F(2) = min([max_force; -k * (position(2)-yWall_L)]);
    end
else
    F(2)=0 ;
end

%Z-walls
if (position(3)<zWall_D)
    if(speed(3) < 0)
        F(3) = min([max_force; -k * (position(3)-zWall_D) + bforward * speed(3)]);
    else
        F(3) = min([max_force; -k * (position(3)-zWall_D)]);
    end
elseif (position(3)>zWall_U)
    if(speed(3) > 0)
        F(3) = max([-max_force; -k * (position(3)-zWall_U) + bforward * speed(3)]);
    else
        F(3) = max([-max_force; -k * (position(3)-zWall_U)]);
    end
else
    F(3)=0;
end

T=F+Fzac;

== matlab function Project_VirtualWall_V7/cooperative position ==
  data: pos_1 input; pos_2 input; circle_pos output; circle_angle output; circle_size output
function [circle_pos,circle_angle,circle_size] = control(pos_1,pos_2)  
    %pos_1 and 2 are the vectors with the x z y positions of the players,
    %circle_angle is in radians cause why not
    % i am assuming pos_2 is the one who starts on the right
    pos_1_yz=pos_1([2 3]);
    pos_2_yz=pos_2([2 3]);
    circle_pos=[0.21;(pos_1(2)+pos_2(2))/2;(pos_1(3)+pos_2(3))/2]; %vector of dimension 3
    pos_aux=pos_2_yz-pos_1_yz;
    circle_size=norm(pos_aux);
    circle_angle=atan2(pos_aux(2),pos_aux(1));

== matlab function Project_VirtualWall_V7/Stena 1 ==
  data: position input; speed input; T output
function T  = control(position, speed)

F= [0; 0; 0];
%Fzac = [0; 0; 0];

%ref pozicija in ravnina
ref_pos=[0.21; 0; -0.21];
Fzac = ([600; 0; 0].*(ref_pos-position)) - ([10; 3; 3].*(speed));


%F= k(ps-pp)-bv

yWall_R = 0.15;
yWall_L = -0.15;
zWall_U = 0.15;
zWall_D = -0.15;

k=1500;
bforward=10;
max_force=25;
%Y-Walls
if (position(2)>yWall_R)
    if(speed(2) > 0)
        F(2) = max([-max_force; -k * (position(2)-yWall_R) + bforward * speed(2)]);
    else
        F(2) = max([-max_force; -k * (position(2)-yWall_R)]);
    end
elseif (position(2)<yWall_L)
    if(speed(2) < 0)
        F(2) = min([max_force; -k * (position(2)-yWall_L) + bforward * speed(2)]);
    else
        F(2) = min([max_force; -k * (position(2)-yWall_L)]);
    end
else
    F(2)=0 ;
end

%Z-walls
if (position(3)<zWall_D)
    if(speed(3) < 0)
        F(3) = min([max_force; -k * (position(3)-zWall_D) + bforward * speed(3)]);
    else
        F(3) = min([max_force; -k * (position(3)-zWall_D)]);
    end
elseif (position(3)>zWall_U)
    if(speed(3) > 0)
        F(3) = max([-max_force; -k * (position(3)-zWall_U) + bforward * speed(3)]);
    else
        F(3) = max([-max_force; -k * (position(3)-zWall_U)]);
    end
else
    F(3)=0;
end

T=F+Fzac;

== matlab function Project_VirtualWall_V7/Collision  ==
  data: cir input; Fadded output; walls output; output_walls output; output_array output; col_variable output; level_flag input
function [Fadded,walls,output_walls,output_array,col_variable]  = All_Walls(cir, level_flag)%position, speed, 

%--------------------------------------------------------------------
%AUTHOR: JAN RAKAR
%DATE  :  4.4.2024
%--------------------------------------------------------------------
%INPUTS
%prevTorque = []         %x, y, radij, rotation
%position                %POSITION OF CENTER SPHERE
%Speed1                   %SPEED OF BOTH PLAYERS
%Speed2
%cir                     %CIRCLE PARAMETER 
%OUTPUTS 
%force added to P1 and P2 (separate forces)
% ----------------------------READDD--------------------------------
% TO DO :
%            ADD force cap
%            WHEN USING THIS AS A FUNCTION UNCOMMENT: %circle = [cir(1), cir(2), cir(3), 0] 

%INPUTS
%cir parameter that contains circle data
%OPTIONAL INPUTS : PLAYER SPEEDS (might add damping later)

%OUTPUT
%force column vector that is generated by all collisions

%cir naj je difajnan kot
%center x, y, radij
%circle = [0,0,1];

%--------VARIABLES--------
k=500;
bforward=10;
max_force=15;
walls = [10 10 0 0;
         10 10 0 0;
         10 10 0 0;
         10 10 0 0;
         10 10 0 0;
         10 10 0 0;
         10 10 0 0;
         10 10 0 0;
         10 10 0 0;
         10 10 0 0;
         10 10 0 0;
         10 10 0 0;
         10 10 0 0;
         10 10 0 0;
         10 10 0 0;
         10 10 0 0];

if (level_flag == 0) 
%x y width(x axis) length(y axis)
    walls = [-0.25 0.25 0.5 0.1;
         0.15 0.25 0.3 0.5;
         -0.15 -0.15 0.5 0.1;
         -0.25 0.25 0.1 0.5;
         -0.05 0.05 0.05 0.25;
         0.05 0.20 0.05 0.25;
         10 10 0 0;
         10 10 0 0;
         10 10 0 0;
         10 10 0 0;
         10 10 0 0;
         10 10 0 0;
         10 10 0 0;
         10 10 0 0;
         10 10 0 0;
         10 10 0 0];
elseif (level_flag == 1)
    walls = [-0.25 0.25 0.5 0.1;
         0.15 0.25 0.3 0.5;
         -0.15 -0.15 0.5 0.1;
         -0.25 0.25 0.1 0.5;
         -0.2 0.1 0.27 0.05;
         0.05 0.2 0.05 0.3;
         -0.1 0 0.1 0.05;
         -0.05 -0.025 0.05 0.12;
         10 10 0 0;
         10 10 0 0;
         10 10 0 0;
         10 10 0 0;
         10 10 0 0;
         10 10 0 0;
         10 10 0 0;
         10 10 0 0];
end
%ADD OUTER WALLS AS THE LAST 4 ROWS
    % -0.25 0.25 0.5 0.1 WHITE ON PIC
    %
    %
    %
    
    
%-0.2 -0.1 0.1 0.1;
%         0.1 0.2 0.1 0.1;
%         0.1 -0.1 0.1 0.1;
         
%debug_col = [0 0 0 0 0 0 0 0 0 0 0 0 0 0 0 0];
col_variable = 0;
output_array = [-2 -2 -2];
closest = [0 0];

Fadded = [0;0;0];
%feed circle data     -> 4th parameter is rotation
circle = [cir(1), cir(2), cir(3)/2, 0] ;
R=circle(3);

%check collision for all walls
[m, n] = size(walls);
for i = 1:m
    %top left corner(x,y) width length
    rect = [walls(i,1),walls(i,2),walls(i,3),walls(i,4)];
    %[col,diff,closest] = CheckCollision(circle, rect);
    %----------------------------------------------------------------
    % Calculate center point of the circle
    circleCenter = [circle(1), circle(2)];

    % Calculate AABB info (center, half-extents)
    rectHalfWidth = rect(3) / 2;
    rectHalfLength = rect(4) / 2;
    rectCenter = [rect(1) + rectHalfWidth, rect(2) - rectHalfLength];

    % Get difference vector between circle center and rectangle center
    difference = circleCenter - rectCenter; %od rect do circ

    % Clamp the difference vector to AABB half-extents
    %OLD APPROACH
    %clampedX = max(-rectHalfWidth, min(difference(1), rectHalfWidth));
    %clampedY = max(-rectHalfLength, min(difference(2), rectHalfLength));%difference je negativen in ga vedno vrne
    %NEW APPROACH
    clampedX = min(abs(difference(1)), abs(rectHalfWidth));
    clampedY = min(abs(difference(2)), abs(rectHalfLength));
    
    if ((rectCenter(1) < circleCenter(1)) && (rectCenter(2) < circleCenter(2)))
        closest = rectCenter + [clampedX, clampedY];
    elseif ((rectCenter(1) < circleCenter(1)) && (rectCenter(2) > circleCenter(2)))
        closest = rectCenter + [clampedX, -clampedY];
    elseif((rectCenter(1) > circleCenter(1)) && (rectCenter(2) > circleCenter(2)))
        closest = rectCenter + [-clampedX, -clampedY];
    elseif((rectCenter(1) > circleCenter(1)) && (rectCenter(2) < circleCenter(2)))
        closest = rectCenter + [-clampedX, +clampedY];
    end
    
    % Add clamped value to rectangle center to get the point on the rectangle closest to the circle
    %closest = rectCenter + [clampedX, clampedY];

    % Check if the closest point is inside the rectangle
    %THIS WAS CHANGED
    %closest(1) = min(max(closest(1), rect(1)), rect(1) + rect(3)); % Clamp x-coordinate
    %closest(2) = min(max(closest(2), rect(2)), rect(2)- rect(4) ); % Clamp y-coordinate
    
    if (i==1)
        output_array(2) = closest(1);
        output_array(3) = closest(2);
    end 
    
    % Retrieve vector between circle center and closest point on rectangle
    difference = closest - circleCenter;
    
    % Check if length of difference vector is less than circle radius
    collision = norm(difference) < circle(3); %%% why is it dependent on R %%%
    
    col = collision;
    diff = difference;
    %[col,diff,closest]
    %[collision,difference,closest]
    %----------------------------------------------------------------
     
    %if collision is detected apply force
    if (col)
        col_variable = 1; 
         %normaliziraj diff vector da postane unit vector
        diff_magnitude = norm(diff);       
        diff_unit = (diff/diff_magnitude) * (-1);     %THIS PARAMETER TELLS YOU WHERE THE VECTOR POINTS%MULTIPLY DIFF BY -1 SO THE VECTOR POINTS IN THE CORRECT DIRECTION
    
        %test = R - hypot(diff(1),diff(2))
        koef = (R - hypot(diff(1),diff(2))) * diff_unit;
        koef = k * koef;
        
        %NOTE: DAMPING CAN BE ADDED LATER
        
        Fadded(2) = Fadded(2) + (koef(1) );    %Y-axis of robot
        Fadded(3) = Fadded(3) + (koef(2) );    %Z-axis of robot
        
    end
    
end


%OUTPUT -> FORCE GENERATED BY ALL COLLISIONS
Fadded = min(max(Fadded, -10), 10);
output_array(1) = col_variable;

%Raztegni walls
output_walls = [walls(1,:) walls(2,:) walls(3,:) walls(4,:) walls(5,:) walls(6,:) walls(7,:) walls(8,:) walls(9,:) walls(10,:) walls(11,:) walls(12,:) walls(13,:) walls(14,:) walls(15,:) walls(16,:)];

end
% %COLLISION FUNCTION
% function [collision,difference,closest] = CheckCollision(circle, rect)
%     
% 
% end

== matlab function Project_VirtualWall_V7/Start_enable  ==
  data: pos1 input; pos2 input; SET output; RESET output; circle input; start_point output; end_point output; startEndPoint output; in input
function [SET, RESET, start_point, end_point, startEndPoint]  = control(pos1, pos2, circle, in)

start_pos= [-0.1, -0.1]; %%z,y,rot so it can be used for end logic
end_pos= [0.125, 0.125]; %%z,y,rot for end
%circle_out = [circle_pos(1),circle_pos(2),circle_size,circle_angle];

distance = 0.008; %allowable distance from start/endpoint
start_radius = 0.04;
start_angle = 1;
angle_tol = 0.08;
%end
end_radius = 0.03;
end_angle = 2;
end_radius2 = 0.03;
end_angle2 = 2;

SET=0;
RESET=0;

start_point = [start_pos(1), start_pos(2), start_radius, start_angle];
end_point = [end_pos(1), end_pos(2), end_radius, end_angle];
startEndPoint = [0 0 0 0];

%%start logic
circle_pos = circle([1 2]);
%start2 = start_pos([1 2]);
if (norm(start_pos - circle_pos) <= distance )
    if (circle(3) < start_radius)
        if (abs(circle(4)-start_angle) < angle_tol)
        SET=1;
        
        end
    end
end

%end logic
if (norm(end_pos - circle_pos) <= distance )
    if (circle(3) < end_radius)
        if (abs(circle(4)-end_angle) < angle_tol)
        %F_enable_latch=0;
        RESET=1;
        
        end
    end
end

if (in == 0)
    startEndPoint = start_point;
elseif(in == 1)
    startEndPoint = end_point;
end

== matlab function Project_VirtualWall_V7/Collision 1 ==
  data: out input; in output
function in    = negator(out)
out = 0;
out = ~in ;
end
% %COLLISION FUNCTION
% function [collision,difference,closest] = CheckCollision(circle, rect)
%     
% 
% end
